simulink model "DroneSimModel_TeamAlpha"  (R2020b)
settings: Solver=VariableStepAuto  StartTime=0.0  StopTime=1800  RelTol=1e-3
libraries: sim3dcameralib x1, sim3dphyssensorlib x1, vehdynlibsens x1, autolibdatasheetbattery x1, shared6dof x1
settings Model: Creator=adamm  LastModifiedBy=jbmic

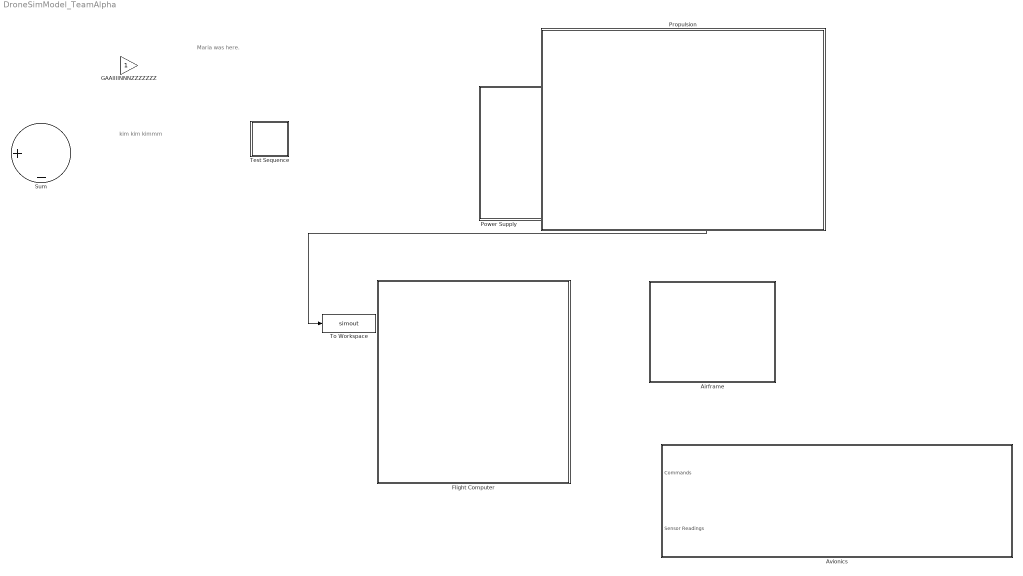
== system DroneSimModel_TeamAlpha ==
  note: kim kim kimmm
  note: Maria was here.
  "Airframe " : Subsystem
  "Avionics " : Subsystem
  "Flight Computer " : Subsystem
  GAAIIIINNNZZZZZZZ : Gain
  "Power Supply " : Subsystem
  "Propulsion " : Subsystem
  Sum : Sum  Inputs=|+-
  Test Sequence : Test Sequence  TreatAsAtomicUnit=on
  To Workspace : ToWorkspace  VariableName=simout  SaveFormat=Timeseries  SampleTime=-1
  wires:
  "Power Supply "/1("Info ") -> To Workspace/1

== system DroneSimModel_TeamAlpha/Airframe  ==

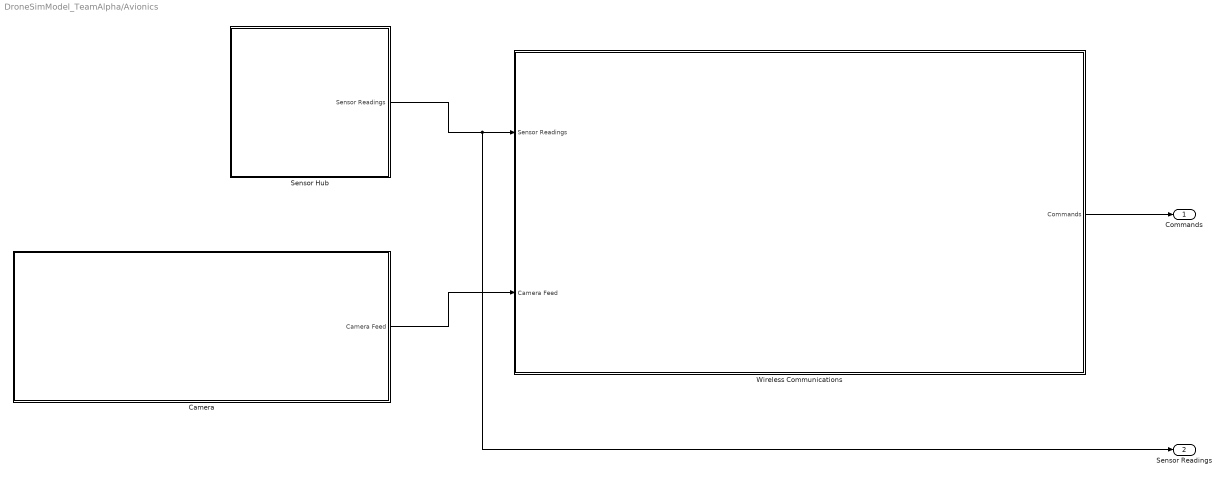
== system DroneSimModel_TeamAlpha/Avionics  ==
  Camera : Subsystem
  Sensor Hub : Subsystem
  Wireless Communications : Subsystem
  "Commands " : Outport
  Sensor Readings : Outport  Port=2
  wires:
  Camera/1(Camera Feed) -> Wireless Communications/2(Camera Feed)
  Sensor Hub/1("Sensor Readings ") -> Wireless Communications/1(Sensor Readings), Sensor Readings/1
  Wireless Communications/1("Commands ") -> "Commands "/1

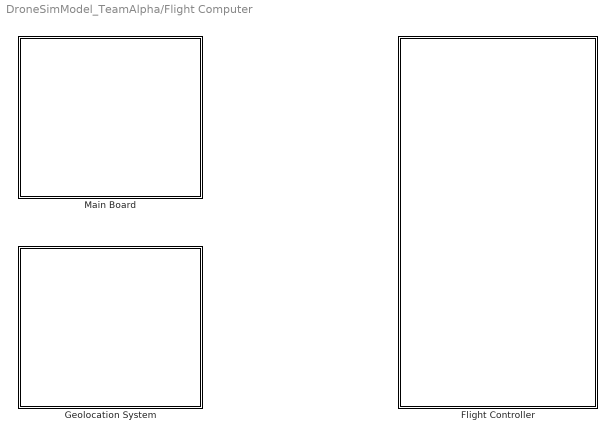
== system DroneSimModel_TeamAlpha/Flight Computer  ==
  "Flight Controller " : Subsystem
  "Geolocation System " : Subsystem
  "Main Board " : Subsystem

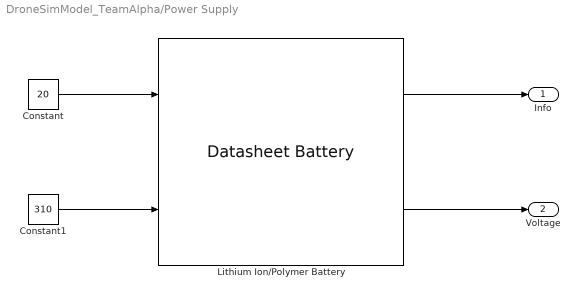
== system DroneSimModel_TeamAlpha/Power Supply  ==
  Constant : Constant  Value=20
  Constant1 : Constant  Value=310
  Lithium Ion/Polymer Battery : autolibdatasheetbattery/Datasheet Battery  CapacityCtrl=Parameter  OutputVlt=Unfiltered  BattChargeMax=10  Em=[2.8 3.228 3.284 3.361 3.408 3.427 3.472 3.477 3.493 3.504 3.516 3.528 3.537 3.545 3.555 3.561 3.566 3.576 3.587 3.589 3.594 3.6 3.608 3.61 3.616 3.619 3.626 3.632 3.637 3.64 3.645 3.646 3.652 3.655 3.658 3.661 3.664 3.668 3.673 3.678 3.68 3.681 3.686 3.692 3.699 3.702 3.705 3.71 3.717 3.723 3.728 3.733 3.735 3.742 3.749 3.755 3.761 3.768 3.773 3.78 3.791 3.798 3.798 3.814 3.818 3.825 3.841 3.846 3.855 3.863 3.877 3.885 3.894 3.907 3.919 3.926 3.935 3.944 3.954 3.964 3.974 3.988 3.998 4.014 4.029 4.034 4.047 4.065 4.074 4.086 4.097 4.131 4.126 4.138 4.15 4.18 4.174 4.187 4.207 4.231 4.221]  CapLUTBp=[0 0.01 0.02 0.03 0.04 0.05 0.06 0.07 0.08 0.09 0.1 0.11 0.12 0.13 0.14 0.15 0.16 0.17 0.18 0.19 0.2 0.21 0.22 0.23 0.24 0.25 0.26 0.27 0.28 0.29 0.3 0.31 0.32 0.33 0.34 0.35 0.36 0.37 0.38 0.39 0.4 0.41 0.42 0.43 0.44 0.45 0.46 0.47 0.48 0.49 0.5 0.51 0.52 0.53 0.54 0.55 0.56 0.57 0.58 0.59 0.6 0.61 0.62 0.63 0.64 0.65 0.66 0.67 0.68 0.69 0.7 0.71 0.72 0.73 0.74 0.75 0.76 0.77 0.78 0.79 0.8 0.81 0.82 0.83 0.84 0.85 0.86 0.87 0.88 0.89 0.9 0.91 0.92 0.93 0.94 0.95 0.96 0.97 0.98 0.99 1]  RInt=[0.008846 0.009319 0.009027 0.00847 0.01032 0.01314;0.006389 0.006554 0.005553 0.005525 0.006043 0.007805;0.004364 0.004101 0.00406 0.003452 0.003846 0.004517;0.002031 0.002563 0.002532 0.00246 0.002716 0.003047;0.001443 0.001825 0.001795 0.001778 0.001924 0.002234;0.0005603 0.0007192 0.0006887 0.0007557 0.0007355 0.001014;0.001028 0.001338 0.001 0.001536 0.001546 0.002789]  BattTempBp=[243.1 253.1 263.1 273.1 283.1 298.1 313.1]  CapSOCBp=[0 0.2 0.4 0.6 0.8 1]  Ns=1  Np=1  BattCapInit=10  Tc=1/1000  Vinit=4.221  RefBlkName='autolibdatasheetbattery/Datasheet Battery'
      settings: SourceProductBaseCode=PW
  "Info " : Outport
  Voltage : Outport  Port=2  OutMin=0  OutMax=12
  wires:
  Constant/1 -> Lithium Ion/Polymer Battery/1
  Constant1/1 -> Lithium Ion/Polymer Battery/2
  Lithium Ion/Polymer Battery/1 -> "Info "/1
  Lithium Ion/Polymer Battery/2 -> Voltage/1

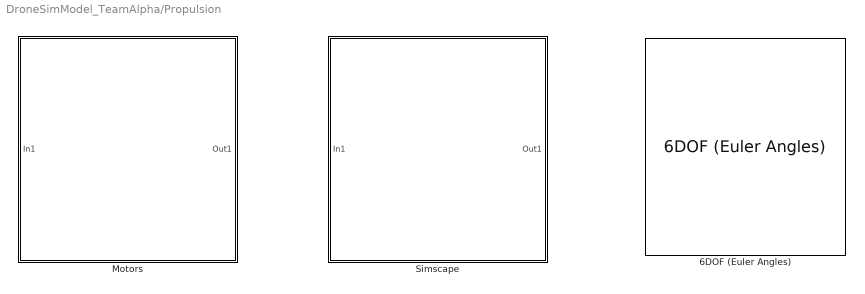
== system DroneSimModel_TeamAlpha/Propulsion  ==
  6DOF (Euler Angles) : shared6dof/6DOF (Euler Angles)  units=Metric (MKS)  mtype=Fixed  rep=Euler Angles  xme_0=[0 0 0]  Vm_0=[0 0 0]  eul_0=[0 0 0]  pm_0=[0 0 0]  mass_0=1.0  mass_e=0.5  mass_f=2.0  inertia=eye(3)  inertia_e=eye(3)  inertia_f=2*eye(3)  k_quat=1.0  vre_flag=on  abi_flag=off  aMode=0  xme_statename=''  Vm_statename=''  eul_statename=''  quat_statename=''  pm_statename=''  mass_statename=''
      settings: SourceProductBaseCode=AE,PW,MT,UV,VE,VP
  "Motors " : Subsystem
  Simscape : Subsystem

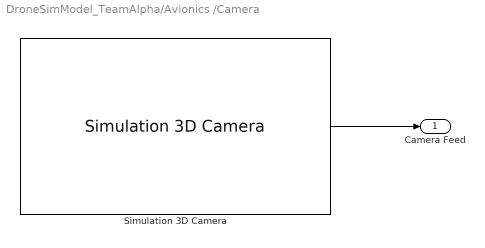
== system DroneSimModel_TeamAlpha/Avionics /Camera ==
  Simulation 3D Camera : sim3dcameralib/Simulation 3D Camera  Priority=1  sensorTag=Sim3dSensor1  sensorId=1  sensorName=Sim3dSensor1  vehTagList={'Scene Origin'}  vehTag=Scene Origin  mountLoc=Origin  offsetFlag=on  tmountOffset=[0, 0, 0]  rmountOffset=[0, 0, 0]  FocalLength=[1109, 1109]  OpticalCenter=[640, 360]  ImageSize=[720, 1280]  RadialDistortion=[0, 0]  TangentialDistortion=[0, 0]  SensorSkew=0  DepthOutportEnabled=off  SemanticOutportEnabled=off  TransformOutportEnabled=off  SampleTime=-1  mountPoint=[0 0 0]  mountOrientation=[0 0 0]  aMode=4  ID=1
      settings: SourceProductBaseCode=DR,UV,VE
  Camera Feed : Outport
  wires:
  Simulation 3D Camera/1 -> Camera Feed/1

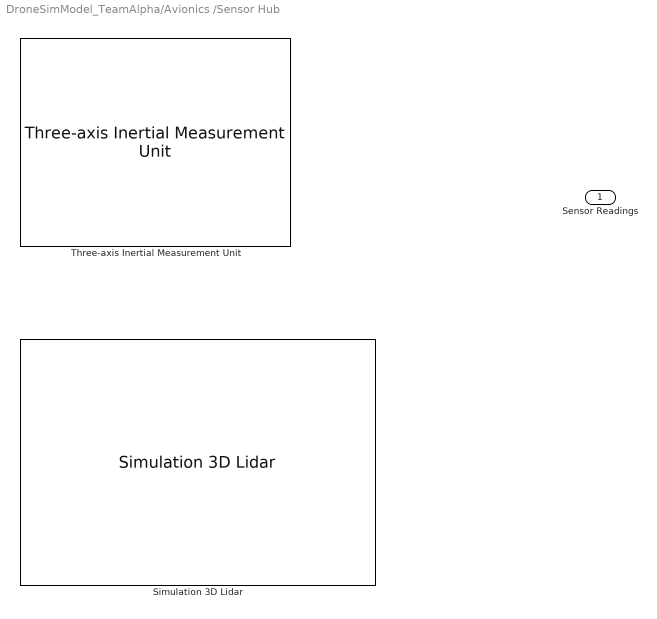
== system DroneSimModel_TeamAlpha/Avionics /Sensor Hub ==
  Simulation 3D Lidar : sim3dphyssensorlib/Simulation 3D Lidar  Priority=1  sensorTag=Sim3dSensor2  sensorId=2  sensorName=Sim3dSensor2  vehTagList={'Scene Origin'}  vehTag=Scene Origin  mountLoc=Origin  offsetFlag=off  tmountOffset=[0, 0, 0]  rmountOffset=[0, 0, 0]  DetectionRange=120  RangeResolution=0.002  VerticalFOV=40  VerticalResolution=1.25  HorizontalFOV=360  HorizontalResolution=0.16  DistanceOutportEnabled=off  TransformOutportEnabled=off  SampleTime=-1  mountPoint=[0 0 0]  mountOrientation=[0 0 0]  aMode=3  ID=2
      settings: SourceProductBaseCode=DR,UV,VE
  Three-axis Inertial Measurement Unit : vehdynlibsens/Three-axis Inertial Measurement Unit  units=Metric (MKS)  imu=[0 0 0]  i_Ts=0  dtype_a=on  w_a=190  z_a=0.707  a_sf_cc=[1 0 0; 0 1 0; 0 0 1]  a_bias=[0 0 0]  a_sat="[-inf  -inf  -inf  inf inf inf]"  dtype_g=on  w_g=190  z_g=0.707  g_sf_cc=[1 0 0; 0 1 0; 0 0 1]  g_bias=[0 0 0]  g_sens=[0 0 0]  g_sat="[-inf  -inf  -inf  inf inf inf]"  i_rand=on  i_seeds=[23093 23094 23095 23096 23097 23098]  i_pow=[0.001 0.001 0.001 0.0001 0.0001 0.0001]  aMode=2
      settings: SourceProductBaseCode=VE
  "Sensor Readings " : Outport

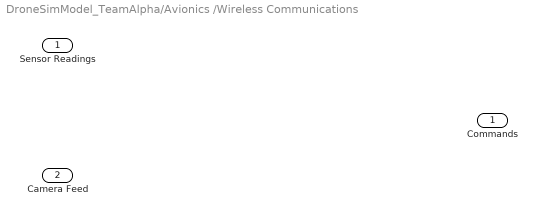
== system DroneSimModel_TeamAlpha/Avionics /Wireless Communications ==
  Sensor Readings : Inport
  Camera Feed : Inport  Port=2
  "Commands " : Outport

== system DroneSimModel_TeamAlpha/Flight Computer /Flight Controller  ==

== system DroneSimModel_TeamAlpha/Flight Computer /Geolocation System  ==

== system DroneSimModel_TeamAlpha/Flight Computer /Main Board  ==

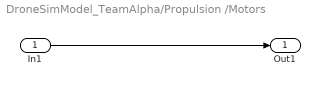
== system DroneSimModel_TeamAlpha/Propulsion /Motors  ==
  In1 : Inport
  Out1 : Outport
  wires:
  In1/1 -> Out1/1

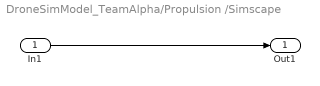
== system DroneSimModel_TeamAlpha/Propulsion /Simscape ==
  In1 : Inport
  Out1 : Outport
  wires:
  In1/1 -> Out1/1

== stateflow chart DroneSimModel_TeamAlpha/Test Sequence ==
  settings: stateMachineType=SIMPLIFIED_MACHINE
  state step_1
  state step_2
  (default) -> step_1
  step_1 -> step_2
